simulink model "mafile"  (R2012b)
settings: Solver=ode45  StartTime=0.0  StopTime=0  RelTol=1e-3
libraries: xbsIndex_r4 x20
settings Model: Creator=abs105  LastModifiedBy=abs105

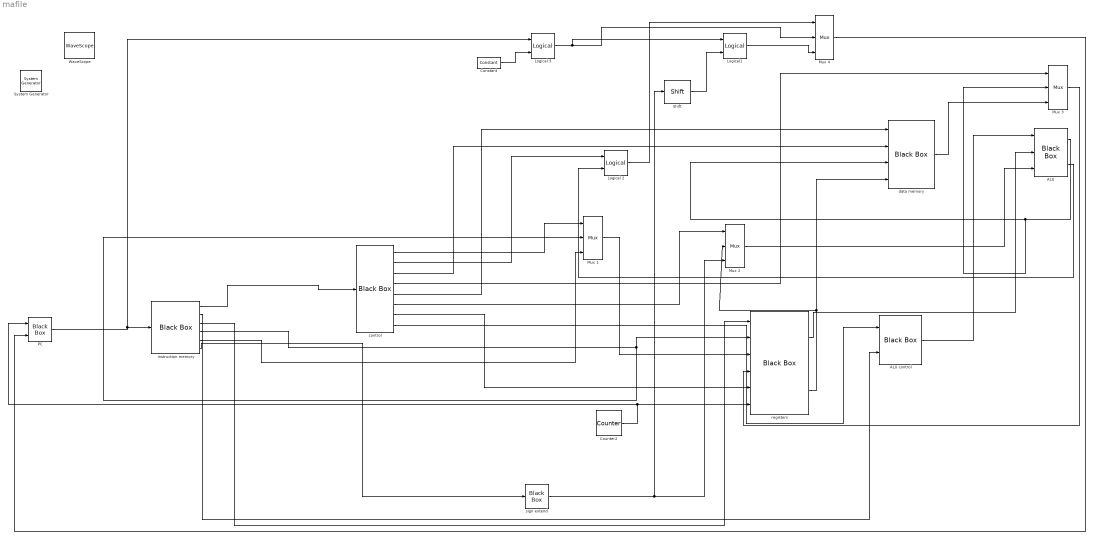
== system mafile ==
  " System Generator" : xbsIndex_r4/ System Generator  Tag=genX  xilinxfamily=Kintex7  part=xc7k325t  speed=-3  package=fbg676  synthesis_tool=XST  clock_wrapper=Clock Enables  directory=./netlist  proj_type=Project Navigator  Synth_file=XST Defaults  Impl_file=ISE Defaults  testbench=off  simulink_period=1  sysclk_period=10  dcm_input_clock_period=10  incr_netlist=off  trim_vbits=Everywhere in SubSystem  dbl_ovrd=According to Block Masks  core_generation=According to Block Masks  run_coregen=off  deprecated_control=off  eval_field=0  block_type=sysgen
  ALU : xbsIndex_r4/Black Box  init_code=alu_config  sim_method=ISE Simulator  verbose=off  block_type=blackbox2
  ALU control : xbsIndex_r4/Black Box  init_code=alucontrol_config  sim_method=ISE Simulator  verbose=off  block_type=blackbox2
  Constant : xbsIndex_r4/Constant  const=4  gui_display_data_type=Fixed-point  arith_type=Unsigned  n_bits=16  bin_pt=0  preci_type=Single  exp_width=8  frac_width=24  explicit_period=on  period=1  equ=P=C  opselect=C  inp2=PCIN>>17  opr=+  inp1=P  carry=CIN  dbl_ovrd=off  block_type=constant
  Counter2 : xbsIndex_r4/Counter  cnt_type=Free Running  cnt_to=Inf  operation=Up  start_count=0  cnt_by_val=1  arith_type=Unsigned  n_bits=1  bin_pt=0  load_pin=off  rst=off  en=off  explicit_period=on  period=1  dbl_ovrd=off  use_behavioral_HDL=off  implementation=Fabric  block_type=counter
  Logical 2 : xbsIndex_r4/Logical  logical_function=AND  inputs=2  en=off  latency=0  precision=Full  arith_type=Unsigned  n_bits=16  bin_pt=0  align_bp=on  dbl_ovrd=off  block_type=logical
  Logical 3 : xbsIndex_r4/Logical  logical_function=AND  inputs=2  en=off  latency=0  precision=Full  arith_type=Unsigned  n_bits=16  bin_pt=0  align_bp=on  dbl_ovrd=off  block_type=logical
  Logical1 : xbsIndex_r4/Logical  logical_function=AND  inputs=2  en=off  latency=0  precision=Full  arith_type=Unsigned  n_bits=16  bin_pt=0  align_bp=on  dbl_ovrd=off  block_type=logical
  Mux 1 : xbsIndex_r4/Mux  inputs=2  en=off  latency=0  precision=User Defined  arith_type=Unsigned  n_bits=5  bin_pt=0  quantization=Truncate  overflow=Wrap  dbl_ovrd=off  block_type=mux
  Mux 2 : xbsIndex_r4/Mux  inputs=2  en=off  latency=0  precision=User Defined  arith_type=Unsigned  n_bits=32  bin_pt=0  quantization=Truncate  overflow=Wrap  dbl_ovrd=off  block_type=mux
  Mux 3 : xbsIndex_r4/Mux  inputs=2  en=off  latency=0  precision=User Defined  arith_type=Unsigned  n_bits=32  bin_pt=0  quantization=Truncate  overflow=Wrap  dbl_ovrd=off  block_type=mux
  Mux 4 : xbsIndex_r4/Mux  inputs=2  en=off  latency=0  precision=User Defined  arith_type=Unsigned  n_bits=32  bin_pt=0  quantization=Truncate  overflow=Wrap  dbl_ovrd=off  block_type=mux
  PC : xbsIndex_r4/Black Box  init_code=programcounter_config  sim_method=ISE Simulator  verbose=off  block_type=blackbox2
  Shift : xbsIndex_r4/Shift  shift_dir=Left  shift_bits=1  en=off  latency=0  precision=User Defined  arith_type=Unsigned  n_bits=32  bin_pt=0  quantization=Truncate  overflow=Wrap  dbl_ovrd=off  block_type=shift
  WaveScope : xbsIndex_r4/WaveScope  block_type=wavescope
  control : xbsIndex_r4/Black Box  init_code=control_config  sim_method=ISE Simulator  verbose=off  block_type=blackbox2
  data memory : xbsIndex_r4/Black Box  init_code=datamem_config  sim_method=ISE Simulator  verbose=off  block_type=blackbox2
  instruction memory : xbsIndex_r4/Black Box  init_code=instrmemo_config  sim_method=ISE Simulator  verbose=off  block_type=blackbox2
  registers : xbsIndex_r4/Black Box  init_code=registers_config  sim_method=ISE Simulator  verbose=off  block_type=blackbox2
  sign extend : xbsIndex_r4/Black Box  init_code=signextend_config  sim_method=ISE Simulator  verbose=off  block_type=blackbox2
  wires:
  Mux 1/1 -> registers/3
  control/6 -> Mux 2/1
  control/1 -> Mux 1/1
  control/7 -> registers/5
  control/5 -> data memory/1
  control/4 -> Mux 3/1
  data memory/1 -> Mux 3/3
  control/3 -> data memory/2
  control/2 -> Logical 2/1
  control/8 -> ALU control/1
  ALU control/1 -> ALU/1
  registers/1 -> ALU/2
  Mux 2/1 -> ALU/3
  registers/2 -> data memory/4, Mux 2/2
  PC/1 -> Logical 3/1, instruction memory/1
  instruction memory/1 -> control/1
  ALU/2 -> Logical 2/2
  ALU/1 -> data memory/3, Mux 3/2
  Mux 3/1 -> registers/4
  instruction memory/4 -> Mux 1/2, registers/2
  instruction memory/3 -> registers/1
  instruction memory/5 -> Mux 1/3
  sign extend/1 -> Shift/1, Mux 2/3
  instruction memory/6 -> sign extend/1
  instruction memory/2 -> ALU control/2
  Logical 2/1 -> Mux 4/1
  Logical1/1 -> Mux 4/3
  Logical 3/1 -> Logical1/1, Mux 4/2
  Shift/1 -> Logical1/2
  Constant/1 -> Logical 3/2
  Counter2/1 -> registers/6, PC/1
  Mux 4/1 -> PC/2
